simulink model "MultiLoop_mode3"  (Simulink 6.2)
settings: Solver=ode1  SolverMode=SingleTasking  StartTime=0.0  StopTime=72  FixedStep=Ts_base  MaxStep=Ts_base  MinStep=1e-6  RelTol=1e-6
PreLoadFcn:
  | Mode_3_Init
StopFcn:
  | TEplot
values from neighbouring files (symbols this model uses):
  r1_0 = 0.251/Fp_0    (= 0.00251)    [Mode_1_Init.m]    (also in Mode_3_Init.m; Skoge_Mode1_Init.m = 0.00267)
  r4_0 = 9.35/Fp_0    (= 0.0935)    [Mode_1_Init.m]    (also in Mode_3_Init.m; Skoge_Mode1_Init.m = 0.0924)
  Ts_base = 0.0005    [Mode_1_Init.m]    (also in Mode_3_Init.m; Skoge_Mode1_Init.m)
  Ts_save = 0.01    [Mode_1_Init.m]    (also in Mode_3_Init.m; Skoge_Mode1_Init.m)
libraries: TElib x17, simulink x2
settings Model: LastModifiedBy=Neil Ricker
settings DataIOCC: LimitDataPoints=off  LoadInitialState=on  SaveFinalState=on  SaveFormat=Structure  SaveOutput=off  SaveTime=off  SignalLoggingName=sigsOut
settings HardwareCC: TargetUnknown=on

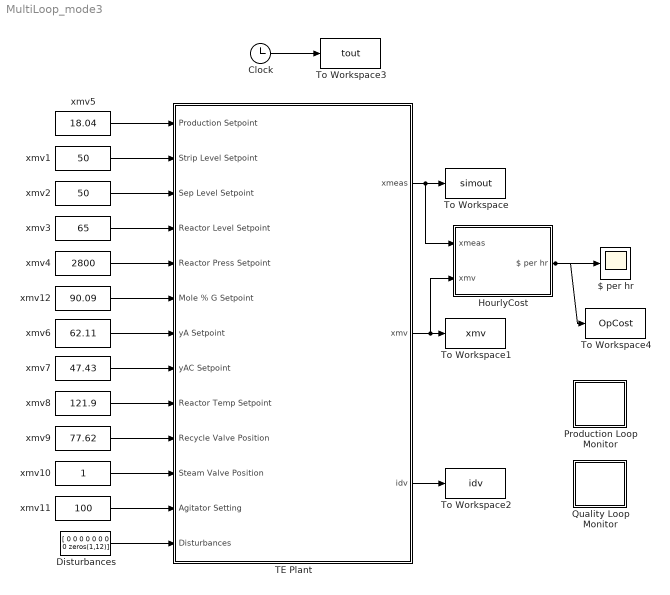
== system MultiLoop_mode3 ==
  $ per hr : Scope
      settings: YMin=25  YMax=275  SaveName=OpCost  DataFormat=Array  SampleInput=on  SampleTime=Ts_save
  Clock : Clock
      settings: Decimation=10
  Disturbances : Constant  Value=[ 0 0 0 0 0 0 0 0 zeros(1,12)]
  HourlyCost : Subsystem
  Production Loop Monitor : Subsystem
  Quality Loop Monitor : Subsystem
  TE Plant : Subsystem
  To Workspace : ToWorkspace  VariableName=simout  SampleTime=Ts_save  SaveFormat=Array
  To Workspace1 : ToWorkspace  VariableName=xmv  SampleTime=Ts_save  SaveFormat=Array
  To Workspace2 : ToWorkspace  VariableName=idv  SampleTime=Ts_save  SaveFormat=Array
  To Workspace3 : ToWorkspace  VariableName=tout  SampleTime=Ts_save  SaveFormat=Array
  To Workspace4 : ToWorkspace  VariableName=OpCost  SampleTime=Ts_save  SaveFormat=Array
  xmv1 : Constant  Value=50
  xmv10 : Constant
  xmv11 : Constant  Value=100
  xmv12 : Constant  Value=90.09
  xmv2 : Constant  Value=50
  xmv3 : Constant  Value=65
  xmv4 : Constant  Value=2800
  xmv5 : Constant  Value=18.04
  xmv6 : Constant  Value=62.11
  xmv7 : Constant  Value=47.43
  xmv8 : Constant  Value=121.9
  xmv9 : Constant  Value=77.62
  wires:
  TE Plant/1(xmeas) -> To Workspace/1, HourlyCost/1(xmeas)
  xmv1/1 -> TE Plant/2(Strip Level Setpoint)
  xmv2/1 -> TE Plant/3(Sep Level Setpoint)
  xmv3/1 -> TE Plant/4(Reactor Level Setpoint)
  xmv4/1 -> TE Plant/5(Reactor Press Setpoint)
  xmv8/1 -> TE Plant/9(Reactor Temp Setpoint)
  xmv6/1 -> TE Plant/7(yA Setpoint)
  xmv7/1 -> TE Plant/8(yAC Setpoint)
  TE Plant/2(xmv) -> To Workspace1/1, HourlyCost/2(xmv)
  TE Plant/3(idv) -> To Workspace2/1
  Clock/1 -> To Workspace3/1
  HourlyCost/1($ per hr) -> $ per hr/1, To Workspace4/1
  xmv9/1 -> TE Plant/10(Recycle Valve Position)
  xmv10/1 -> TE Plant/11(Steam Valve Position)
  xmv11/1 -> TE Plant/12(Agitator Setting)
  Disturbances/1 -> TE Plant/13(Disturbances)
  xmv12/1 -> TE Plant/6(Mole % G Setpoint)
  xmv5/1 -> TE Plant/1(Production Setpoint)

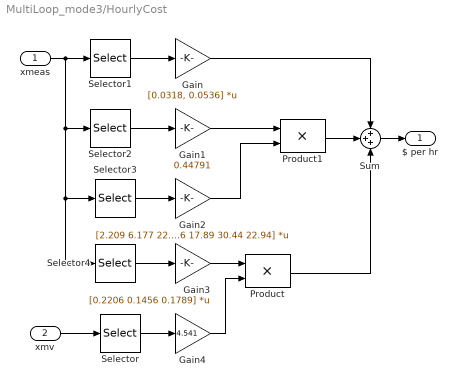
== system MultiLoop_mode3/HourlyCost ==
  xmeas : Inport  Port=1  PortDimensions=41  LatchInput=off
  xmv : Inport  Port=2  PortDimensions=12  LatchInput=off
  Gain : Gain  Gain=[0.0318, 0.0536]  Multiplication=Matrix(K*u)  SaturateOnIntegerOverflow=on
  Gain1 : Gain  Gain=0.44791  SaturateOnIntegerOverflow=on
  Gain2 : Gain  Gain=[2.209 6.177 22.06 14.56 17.89 30.44 22.94]  Multiplication=Matrix(K*u)  SaturateOnIntegerOverflow=on
  Gain3 : Gain  Gain=[0.2206 0.1456 0.1789]  Multiplication=Matrix(K*u)  SaturateOnIntegerOverflow=on
  Gain4 : Gain  Gain=4.541  SaturateOnIntegerOverflow=on
  Product : Product  SaturateOnIntegerOverflow=on
  Product1 : Product  SaturateOnIntegerOverflow=on
  Selector : Selector  Elements=8  InputPortWidth=12
  Selector1 : Selector  Elements=[19 20]  InputPortWidth=41
  Selector2 : Selector  Elements=[10]  InputPortWidth=41
  Selector3 : Selector  Elements=[29, 31:36]  InputPortWidth=41
  Selector4 : Selector  Elements=[37:39]  InputPortWidth=41
  Sum : Sum  Inputs=+++  SaturateOnIntegerOverflow=on
  $ per hr : Outport
  wires:
  xmv/1 -> Selector/1
  xmeas/1 -> Selector1/1, Selector2/1, Selector3/1, Selector4/1
  Selector1/1 -> Gain/1
  Selector2/1 -> Gain1/1
  Selector3/1 -> Gain2/1
  Selector4/1 -> Gain3/1
  Selector/1 -> Gain4/1
  Gain3/1 -> Product/1
  Gain4/1 -> Product/2
  Sum/1 -> $ per hr/1
  Product/1 -> Sum/3
  Gain/1 -> Sum/1
  Product1/1 -> Sum/2
  Gain1/1 -> Product1/1
  Gain2/1 -> Product1/2

== system MultiLoop_mode3/Production Loop Monitor ==
  Mux2 : Mux  Inputs=2
  Production : Scope
      settings: YMin=20  YMax=28  SaveName=Production  SampleInput=on  SampleTime=Ts_save
  wires:
  Mux2/1 -> Production/1
  [xmeas17] -> Mux2/2
  [Prodsp] -> Mux2/1

== system MultiLoop_mode3/Quality Loop Monitor ==
  Mux2 : Mux  Inputs=2
  Quality : Scope
      settings: YMin=40  YMax=60  SaveName=Quality  SampleInput=on  SampleTime=Ts_save
  wires:
  [PctGsp] -> Mux2/1
  [xmeas40] -> Mux2/2
  Mux2/1 -> Quality/1

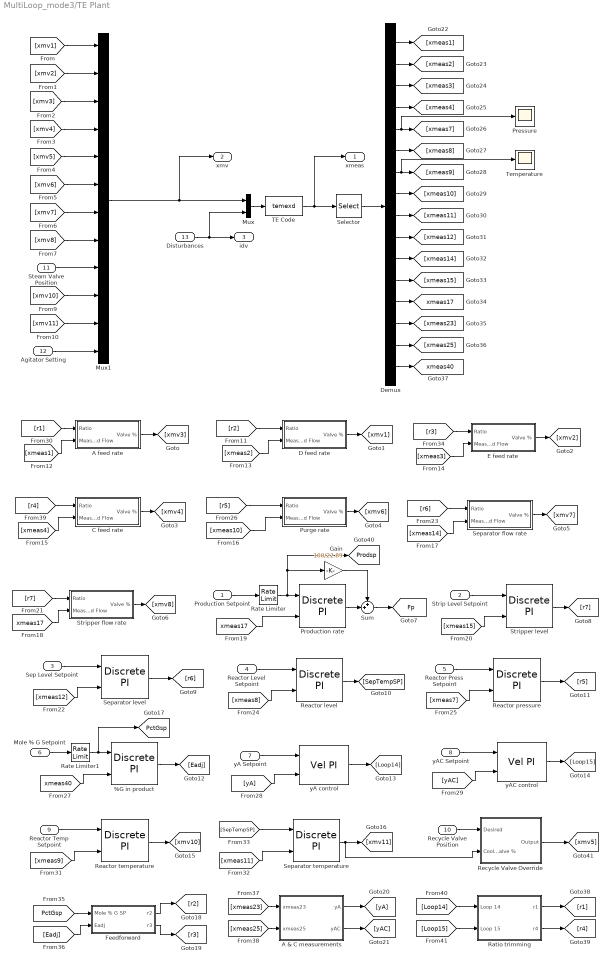
== system MultiLoop_mode3/TE Plant ==
  Production Setpoint : Inport  Port=1  LatchInput=off
  Strip Level Setpoint : Inport  Port=2  LatchInput=off
  Sep Level Setpoint : Inport  Port=3  LatchInput=off
  Reactor Level Setpoint : Inport  Port=4  LatchInput=off
  Reactor Press Setpoint : Inport  Port=5  LatchInput=off
  Mole % G Setpoint : Inport  Port=6  LatchInput=off
  yA Setpoint : Inport  Port=7  LatchInput=off
  yAC Setpoint : Inport  Port=8  LatchInput=off
  Reactor Temp Setpoint : Inport  Port=9  LatchInput=off
  Recycle Valve Position : Inport  Port=10  LatchInput=off
  Steam Valve Position : Inport  Port=11  LatchInput=off
  Agitator Setting : Inport  Port=12  LatchInput=off
  Disturbances : Inport  Port=13  LatchInput=off
  %G in product : TElib/Discrete PI  Kc=-0.4  Ti=100/60  Ts=Ts_base  x0=Eadj_0  Hi=inf  Lo=-inf
  A & C measurements : Subsystem
  A feed rate : Subsystem
  C feed rate : Subsystem
  D feed rate : Subsystem
  Demux : Demux  Outputs=16
  E feed rate : Subsystem
  Feedforward : Subsystem
  Gain : Gain  Gain=100/22.89  SaturateOnIntegerOverflow=on
  Mux : Mux  Inputs=2
  Mux1 : Mux  Inputs=12
  Pressure : Scope
      settings: YMin=2700  YMax=2900  SampleInput=on  SampleTime=Ts_save
  Production rate : TElib/Discrete PI  Kc=3.2  Ti=120/60  Ts=Ts_base  x0=0  Hi=30  Lo=-30
  Purge rate : Subsystem
  Rate Limiter : RateLimiter  RisingSlewLimit=0.3*22.95/24  FallingSlewLimit=-0.3*22.95/24
  Rate Limiter1 : RateLimiter  RisingSlewLimit=50/24  FallingSlewLimit=-50/24
  Ratio trimming : Subsystem
  Reactor level : TElib/Discrete PI  Kc=0.8  Ti=60/60  Ts=Ts_base  x0=SP17_0  Hi=120  Lo=0
  Reactor pressure : TElib/Discrete PI  Kc=-1e-4  Ti=20/60  Ts=Ts_base  x0=r5_0  Hi=100  Lo=0
  Reactor temperature : TElib/Discrete PI  Kc=-8  Ti=7.5/60  Ts=Ts_base  x0=xmv10_0  Hi=100  Lo=0
  Recycle Valve Override : Subsystem  AncestorBlock=TElib/Discrete PI
  Selector : Selector  Elements=[1:4, 7:12, 14, 15, 17, 23, 25, 40]  InputPortWidth=41
  Separator flow rate : Subsystem
  Separator level : TElib/Discrete PI  Kc=-1e-3  Ti=200/60  Ts=Ts_base  x0=r6_0  Hi=100  Lo=0
  Separator temperature : TElib/Discrete PI  Kc=-4  Ti=15/60  Ts=Ts_base  x0=xmv11_0  Hi=100  Lo=0
  Stripper flow rate : Subsystem
  Stripper level : TElib/Discrete PI  Kc=-2e-4  Ti=200/60  Ts=Ts_base  x0=r7_0  Hi=100  Lo=0
  Sum : Sum  Inputs=++|  SaturateOnIntegerOverflow=on
  TE Code : S-Function  FunctionName=temexd  Parameters=[]
  Temperature : Scope
      settings: YMin=120  YMax=130  SampleInput=on  SampleTime=Ts_save
  yA control : TElib/Discrete PI/Vel PI  Kc=2e-4  Ti=1  Ts=0.1
  yAC control : TElib/Discrete PI/Vel PI  Kc=3e-4  Ti=2  Ts=0.1
  xmeas : Outport
  xmv : Outport  Port=2
  idv : Outport  Port=3
  tag scope: Fp=global, PctGsp=global, Prodsp=global, xmeas17=global, xmeas40=global
  wires:
  Mux/1 -> TE Code/1
  Disturbances/1 -> Mux/2, idv/1
  TE Code/1 -> xmeas/1, Selector/1
  [xmv1] -> Mux1/1
  [xmv2] -> Mux1/2
  [xmv3] -> Mux1/3
  [xmv4] -> Mux1/4
  [xmv6] -> Mux1/6
  [xmv7] -> Mux1/7
  [xmv8] -> Mux1/8
  Steam Valve Position/1 -> Mux1/9
  [xmv10] -> Mux1/10
  [xmv11] -> Mux1/11
  Agitator Setting/1 -> Mux1/12
  A feed rate/1(Valve %) -> [xmv3]
  [xmeas1] -> A feed rate/2(Measured Flow)
  D feed rate/1(Valve %) -> [xmv1]
  [xmeas2] -> D feed rate/2(Measured Flow)
  E feed rate/1(Valve %) -> [xmv2]
  [xmeas3] -> E feed rate/2(Measured Flow)
  C feed rate/1(Valve %) -> [xmv4]
  [xmeas4] -> C feed rate/2(Measured Flow)
  Purge rate/1(Valve %) -> [xmv6]
  [xmeas10] -> Purge rate/2(Measured Flow)
  Separator flow rate/1(Valve %) -> [xmv7]
  [xmeas14] -> Separator flow rate/2(Measured Flow)
  Stripper flow rate/1(Valve %) -> [xmv8]
  [xmeas17] -> Stripper flow rate/2(Measured Flow)
  [xmeas17] -> Production rate/2
  [xmeas15] -> Stripper level/2
  Strip Level Setpoint/1 -> Stripper level/1
  Stripper level/1 -> [r7]
  [r7] -> Stripper flow rate/1(Ratio)
  [xmeas12] -> Separator level/2
  Sep Level Setpoint/1 -> Separator level/1
  Separator level/1 -> [r6]
  [r6] -> Separator flow rate/1(Ratio)
  [xmeas8] -> Reactor level/2
  Reactor Level Setpoint/1 -> Reactor level/1
  Reactor level/1 -> [SepTempSP]
  [xmeas7] -> Reactor pressure/2
  Reactor Press Setpoint/1 -> Reactor pressure/1
  Reactor pressure/1 -> [r5]
  [r5] -> Purge rate/1(Ratio)
  [xmeas40] -> %G in product/2
  %G in product/1 -> [Eadj]
  [yA] -> yA control/2
  yA Setpoint/1 -> yA control/1
  yA control/1 -> [Loop14]
  [yAC] -> yAC control/2
  yAC Setpoint/1 -> yAC control/1
  yAC control/1 -> [Loop15]
  [r1] -> A feed rate/1(Ratio)
  [xmeas9] -> Reactor temperature/2
  Reactor Temp Setpoint/1 -> Reactor temperature/1
  Reactor temperature/1 -> [xmv10]
  [xmeas11] -> Separator temperature/2
  [SepTempSP] -> Separator temperature/1
  Separator temperature/1 -> [xmv11], Recycle Valve Override/2(Coolant Valve %)
  [r2] -> D feed rate/1(Ratio)
  [r3] -> E feed rate/1(Ratio)
  [PctGsp] -> Feedforward/1(Mole % G SP)
  [Eadj] -> Feedforward/2(Eadj)
  Feedforward/1(r2) -> [r2]
  Feedforward/2(r3) -> [r3]
  [xmeas23] -> A & C measurements/1(xmeas23)
  [xmeas25] -> A & C measurements/2(xmeas25)
  A & C measurements/1(yA) -> [yA]
  A & C measurements/2(yAC) -> [yAC]
  Mux1/1 -> Mux/1, xmv/1
  Selector/1 -> Demux/1
  Demux/1 -> [xmeas1]
  Demux/2 -> [xmeas2]
  Demux/3 -> [xmeas3]
  Demux/4 -> [xmeas4]
  Demux/5 -> [xmeas7], Pressure/1
  Demux/6 -> [xmeas8]
  Demux/7 -> [xmeas9], Temperature/1
  Demux/8 -> [xmeas10]
  Demux/9 -> [xmeas11]
  Demux/10 -> [xmeas12]
  Demux/11 -> [xmeas14]
  Demux/12 -> [xmeas15]
  Demux/13 -> [xmeas17]
  Demux/14 -> [xmeas23]
  Demux/15 -> [xmeas25]
  Demux/16 -> [xmeas40]
  [r4] -> C feed rate/1(Ratio)
  [Loop14] -> Ratio trimming/1(Loop 14)
  [Loop15] -> Ratio trimming/2(Loop 15)
  Ratio trimming/1(r1) -> [r1]
  Ratio trimming/2(r4) -> [r4]
  Production Setpoint/1 -> Rate Limiter/1
  Rate Limiter/1 -> Production rate/1, [Prodsp], Gain/1
  Mole % G Setpoint/1 -> Rate Limiter1/1
  Rate Limiter1/1 -> %G in product/1, [PctGsp]
  Production rate/1 -> Sum/2
  Sum/1 -> [Fp]
  Gain/1 -> Sum/1
  [xmv5] -> Mux1/5
  Recycle Valve Override/1(Output) -> [xmv5]
  Recycle Valve Position/1 -> Recycle Valve Override/1(Desired)

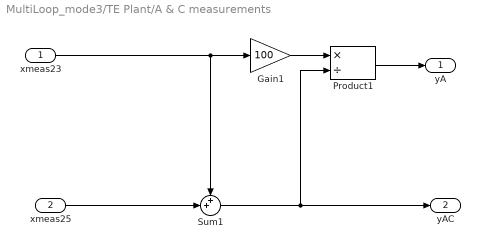
== system MultiLoop_mode3/TE Plant/A & C measurements ==
  xmeas23 : Inport  Port=1  LatchInput=off
  xmeas25 : Inport  Port=2  LatchInput=off
  Gain1 : Gain  Gain=100  SaturateOnIntegerOverflow=on
  Product1 : Product  Inputs=*/  SaturateOnIntegerOverflow=on
  Sum1 : Sum  Inputs=++|  SaturateOnIntegerOverflow=on
  yA : Outport
  yAC : Outport  Port=2
  wires:
  Sum1/1 -> yAC/1, Product1/2
  xmeas23/1 -> Sum1/1, Gain1/1
  xmeas25/1 -> Sum1/2
  Gain1/1 -> Product1/1
  Product1/1 -> yA/1

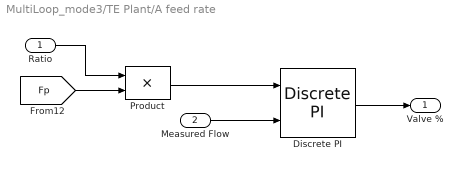
== system MultiLoop_mode3/TE Plant/A feed rate ==
  Ratio : Inport  Port=1  LatchInput=off
  Measured Flow : Inport  Port=2  LatchInput=off
  Discrete PI : TElib/Discrete PI  Kc=0.01  Ti=0.001/60  Ts=Ts_base  x0=xmv3_0  Hi=100  Lo=0
  Product : Product  SaturateOnIntegerOverflow=on
  Valve % : Outport
  wires:
  Discrete PI/1 -> Valve %/1
  Ratio/1 -> Product/1
  [Fp] -> Product/2
  Measured Flow/1 -> Discrete PI/2
  Product/1 -> Discrete PI/1

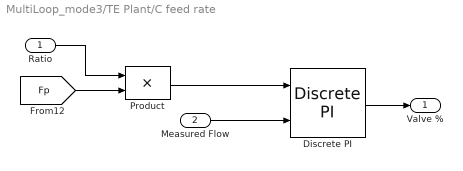
== system MultiLoop_mode3/TE Plant/C feed rate ==
  Ratio : Inport  Port=1  LatchInput=off
  Measured Flow : Inport  Port=2  LatchInput=off
  Discrete PI : TElib/Discrete PI  Kc=0.003  Ti=0.001/60  Ts=Ts_base  x0=xmv4_0  Hi=100  Lo=0
  Product : Product  SaturateOnIntegerOverflow=on
  Valve % : Outport
  wires:
  Product/1 -> Discrete PI/1
  Measured Flow/1 -> Discrete PI/2
  [Fp] -> Product/2
  Ratio/1 -> Product/1
  Discrete PI/1 -> Valve %/1

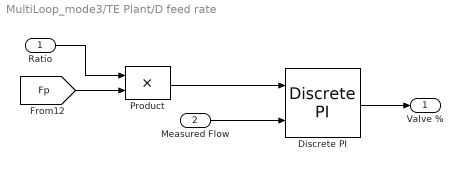
== system MultiLoop_mode3/TE Plant/D feed rate ==
  Ratio : Inport  Port=1  LatchInput=off
  Measured Flow : Inport  Port=2  LatchInput=off
  Discrete PI : TElib/Discrete PI  Kc=1.6e-6  Ti=0.001/60  Ts=Ts_base  x0=xmv1_0  Hi=100  Lo=0
  Product : Product  SaturateOnIntegerOverflow=on
  Valve % : Outport
  wires:
  Product/1 -> Discrete PI/1
  Measured Flow/1 -> Discrete PI/2
  [Fp] -> Product/2
  Ratio/1 -> Product/1
  Discrete PI/1 -> Valve %/1

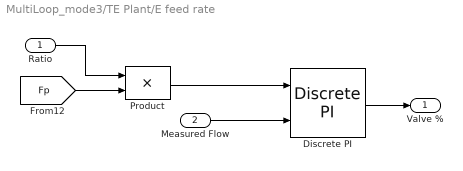
== system MultiLoop_mode3/TE Plant/E feed rate ==
  Ratio : Inport  Port=1  LatchInput=off
  Measured Flow : Inport  Port=2  LatchInput=off
  Discrete PI : TElib/Discrete PI  Kc=1.8e-6  Ti=0.001/60  Ts=Ts_base  x0=xmv2_0  Hi=100  Lo=0
  Product : Product  SaturateOnIntegerOverflow=on
  Valve % : Outport
  wires:
  Product/1 -> Discrete PI/1
  Measured Flow/1 -> Discrete PI/2
  [Fp] -> Product/2
  Ratio/1 -> Product/1
  Discrete PI/1 -> Valve %/1

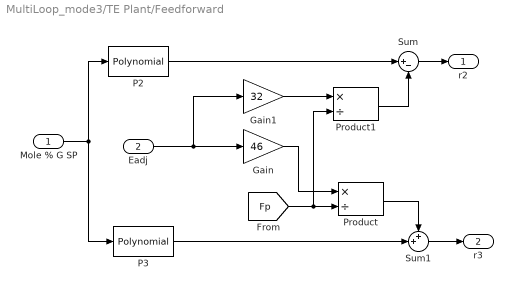
== system MultiLoop_mode3/TE Plant/Feedforward ==
  Mole % G SP : Inport  Port=1  LatchInput=off
  Eadj : Inport  Port=2  LatchInput=off
  Gain : Gain  Gain=46  SaturateOnIntegerOverflow=on
  Gain1 : Gain  Gain=32  SaturateOnIntegerOverflow=on
  P2 : simulink/Math Operations/Polynomial  coefs="[1.5192e-003  5.9446e-001  2.7690e-001]"
  P3 : simulink/Math Operations/Polynomial  coefs="[-1.1377e-003 -8.0893e-001  9.1060e+001]"
  Product : Product  Inputs=*/  SaturateOnIntegerOverflow=on
  Product1 : Product  Inputs=*/  SaturateOnIntegerOverflow=on
  Sum : Sum  Inputs=|+-  SaturateOnIntegerOverflow=on
  Sum1 : Sum  Inputs=++|  SaturateOnIntegerOverflow=on
  r2 : Outport
  r3 : Outport  Port=2
  wires:
  Mole % G SP/1 -> P2/1, P3/1
  Sum/1 -> r2/1
  P2/1 -> Sum/1
  Sum1/1 -> r3/1
  P3/1 -> Sum1/2
  Product/1 -> Sum1/1
  [Fp] -> Product/2, Product1/2
  Gain/1 -> Product/1
  Eadj/1 -> Gain/1, Gain1/1
  Product1/1 -> Sum/2
  Gain1/1 -> Product1/1

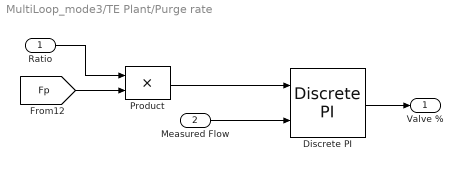
== system MultiLoop_mode3/TE Plant/Purge rate ==
  Ratio : Inport  Port=1  LatchInput=off
  Measured Flow : Inport  Port=2  LatchInput=off
  Discrete PI : TElib/Discrete PI  Kc=0.01  Ti=0.001/60  Ts=Ts_base  x0=xmv6_0  Hi=100  Lo=0
  Product : Product  SaturateOnIntegerOverflow=on
  Valve % : Outport
  wires:
  Discrete PI/1 -> Valve %/1
  Ratio/1 -> Product/1
  [Fp] -> Product/2
  Measured Flow/1 -> Discrete PI/2
  Product/1 -> Discrete PI/1

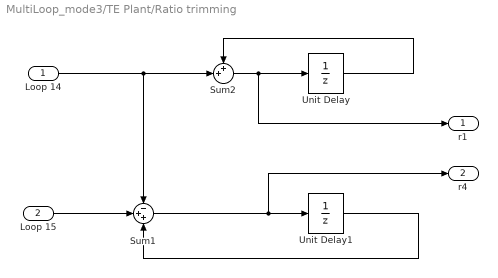
== system MultiLoop_mode3/TE Plant/Ratio trimming ==
  Loop 14 : Inport  Port=1  LatchInput=off
  Loop 15 : Inport  Port=2  LatchInput=off
  Sum1 : Sum  Inputs=-++  SaturateOnIntegerOverflow=on
  Sum2 : Sum  Inputs=++|  SaturateOnIntegerOverflow=on
  Unit Delay : UnitDelay  X0=r1_0  SampleTime=0.1
  Unit Delay1 : UnitDelay  X0=r4_0  SampleTime=0.1
  r1 : Outport
  r4 : Outport  Port=2
  wires:
  Loop 15/1 -> Sum1/2
  Unit Delay/1 -> Sum2/1
  Unit Delay1/1 -> Sum1/3
  Sum2/1 -> Unit Delay/1, r1/1
  Loop 14/1 -> Sum2/2, Sum1/1
  Sum1/1 -> Unit Delay1/1, r4/1

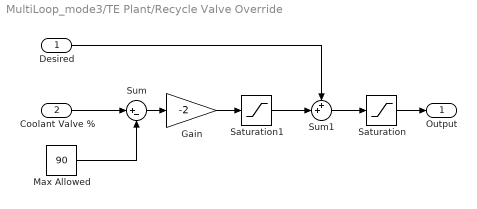
== system MultiLoop_mode3/TE Plant/Recycle Valve Override ==
  Desired : Inport  Port=1  LatchInput=off
  Coolant Valve % : Inport  Port=2  LatchInput=off
  Gain : Gain  Gain=-2
  Max Allowed : Constant  Value=90
  Saturation : Saturate  UpperLimit=100  LowerLimit=0
  Saturation1 : Saturate  UpperLimit=0  LowerLimit=-Inf
  Sum : Sum  Inputs=|+-  SaturateOnIntegerOverflow=on
  Sum1 : Sum  Inputs=++|
  Output : Outport
  wires:
  Saturation/1 -> Output/1
  Coolant Valve %/1 -> Sum/1
  Sum/1 -> Gain/1
  Max Allowed/1 -> Sum/2
  Gain/1 -> Saturation1/1
  Sum1/1 -> Saturation/1
  Saturation1/1 -> Sum1/2
  Desired/1 -> Sum1/1

== system MultiLoop_mode3/TE Plant/Separator flow rate ==
  Ratio : Inport  Port=1  LatchInput=off
  Measured Flow : Inport  Port=2  LatchInput=off
  Discrete PI : TElib/Discrete PI  Kc=4e-4  Ti=0.001/60  Ts=Ts_base  x0=xmv7_0  Hi=100  Lo=0
  Product : Product  SaturateOnIntegerOverflow=on
  Valve % : Outport
  wires:
  Product/1 -> Discrete PI/1
  Measured Flow/1 -> Discrete PI/2
  [Fp] -> Product/2
  Ratio/1 -> Product/1
  Discrete PI/1 -> Valve %/1

== system MultiLoop_mode3/TE Plant/Stripper flow rate ==
  Ratio : Inport  Port=1  LatchInput=off
  Measured Flow : Inport  Port=2  LatchInput=off
  Discrete PI : TElib/Discrete PI  Kc=4e-4  Ti=0.001/60  Ts=Ts_base  x0=xmv8_0  Hi=100  Lo=0
  Product : Product  SaturateOnIntegerOverflow=on
  Valve % : Outport
  wires:
  Discrete PI/1 -> Valve %/1
  Ratio/1 -> Product/1
  [Fp] -> Product/2
  Measured Flow/1 -> Discrete PI/2
  Product/1 -> Discrete PI/1
